simulink model "Dynamics_test1"  (R2021b)
settings: Solver=VariableStepAuto  StartTime=0.0  StopTime=10.0  RelTol=1e-3
InitFcn:
  | % ************** Initiate forces
  | % f0=[0;0;0;0;0;0];
  | % f0=[0;0;0;0;0;0;0];
  | f_0=[0;0;0];
  | f_m=[0;0];
  | f_e=[0;0;0;0;0;0];
  | % ************** Initiate states
  | q_m=[0;0];
  | q_dot_m=[0;0];
  | P=[0;0;0];
  | V_I0=[0;0;0];
  | % ************** Load main
  | %run(Main.m)
values from neighbouring files (symbols this model uses):
  diag_M = diagonalize(M_frak0, M_frak)    [Create_Robot.m]    (also in Main.m; diagonalize.m = zeros(6*(n+1),6*(n+1)); test_C_Main.m)
  iota0 = [1 0 0; 0 1 0;zeros(3,3);0 0 1]    [Create_Robot.m]    (also in Main.m = eye(6,6); test_C_Main.m)
  Xi_m_matrix = zeros(6*n,n)    [Create_Robot.m]    (also in Main.m; test_C_Main.m)
undefined symbols (not defined in the file or in its folder): Xi_m
settings Model: Creator=Bmmog  LastModifiedBy=Bmmog
settings SolverCC: AllowMultiTaskInputOutput=on

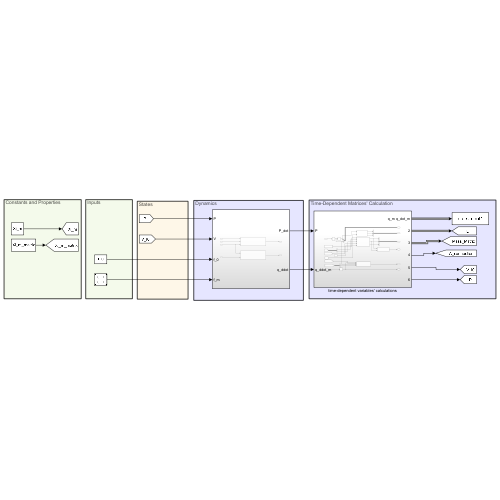
[thumbnail: Simulink's stored preview of the top-level diagram]
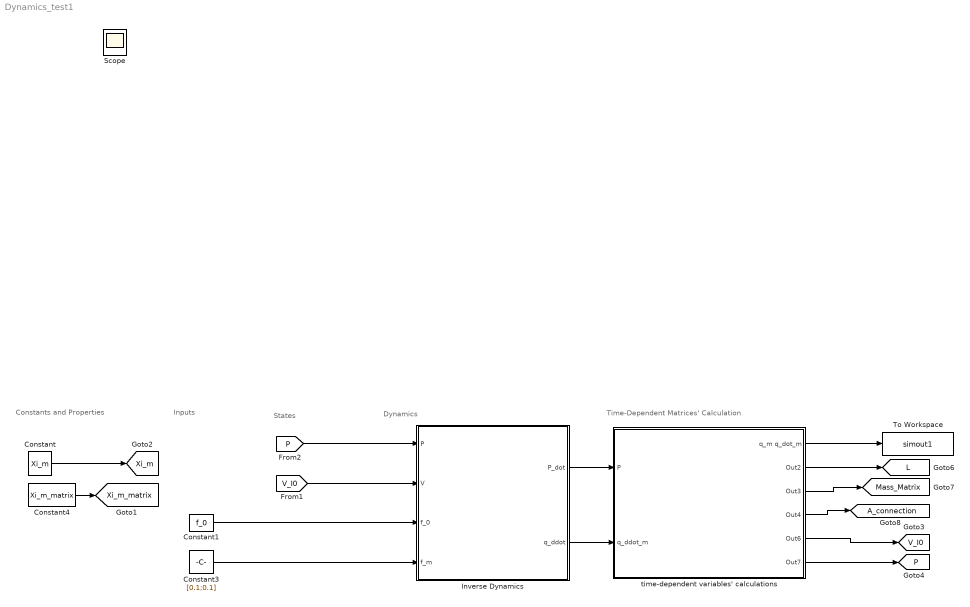
== system Dynamics_test1 ==
  note: Time-Dependent Matrices' Calculation
  note: States
  note: Inputs
  note: Dynamics
  note: Constants and Properties
  Constant : Constant  Value=Xi_m  VectorParams1D=off
  Constant1 : Constant  Value=f_0  VectorParams1D=off
  Constant3 : Constant  Value=[0.1;0.1]  VectorParams1D=off
  Constant4 : Constant  Value=Xi_m_matrix  VectorParams1D=off
  Inverse Dynamics : Subsystem
  To Workspace : ToWorkspace  VariableName=simout1  SaveFormat=Timeseries  SampleTime=-1
  time-dependent variables' calculations : Subsystem
  Scope : Scope
  tag scope: A_connection=global, L=global, Mass_Matrix=global, P=global, V_I0=global, Xi_m=global, Xi_m_matrix=global
  wires:
  Constant/1 -> [Xi_m]
  Constant4/1 -> [Xi_m_matrix]
  Constant1/1 -> Inverse Dynamics/3(f_0)
  Constant3/1 -> Inverse Dynamics/4(f_m)
  [P] -> Inverse Dynamics/1(P)
  [V_I0] -> Inverse Dynamics/2(V)
  time-dependent variables' calculations/6(Out7) -> [P]
  time-dependent variables' calculations/5(Out6) -> [V_I0]
  time-dependent variables' calculations/4(Out4) -> [A_connection]
  time-dependent variables' calculations/3(Out3) -> [Mass_Matrix]
  time-dependent variables' calculations/2(Out2) -> [L]
  time-dependent variables' calculations/1(q_m q_dot_m) -> To Workspace/1
  Inverse Dynamics/1(P_dot) -> time-dependent variables' calculations/1(P)
  Inverse Dynamics/2(q_ddot) -> time-dependent variables' calculations/2(q_ddot_m)

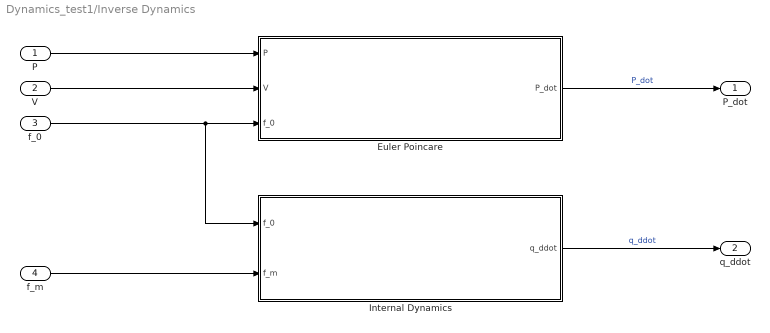
== system Dynamics_test1/Inverse Dynamics ==
  P : Inport
  V : Inport  Port=2
  f_0 : Inport  Port=3
  f_m : Inport  Port=4
  Euler Poincare : Subsystem
  Internal Dynamics : Subsystem
  P_dot : Outport
  q_ddot : Outport  Port=2
  wires:
  f_0/1 -> Internal Dynamics/1(f_0), Euler Poincare/3(f_0)
  f_m/1 -> Internal Dynamics/2(f_m)
  Internal Dynamics/1(q_ddot) -> q_ddot/1  "q_ddot"
  Euler Poincare/1(P_dot) -> P_dot/1  "P_dot"
  P/1 -> Euler Poincare/1(P)
  V/1 -> Euler Poincare/2(V)

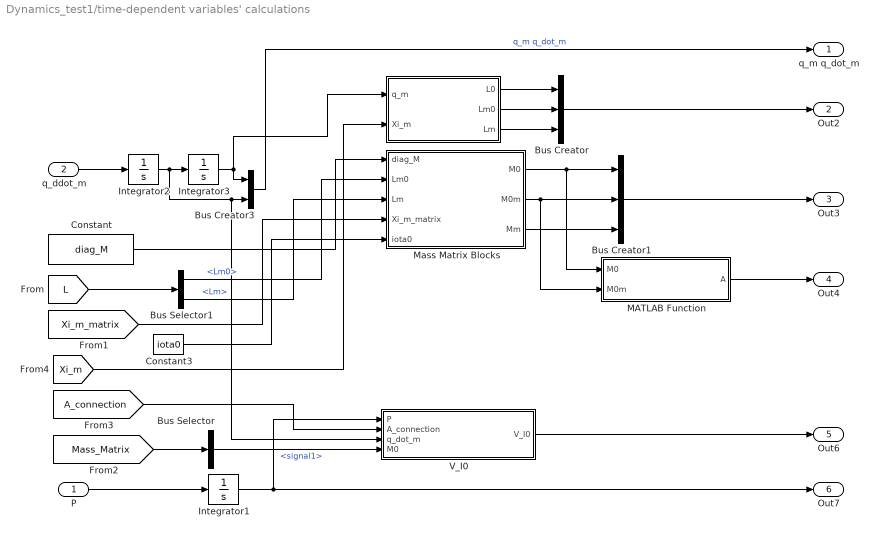
== system Dynamics_test1/time-dependent variables' calculations ==
  P : Inport
  q_ddot_m : Inport  Port=2
  " " : MATLAB Function  TreatAsAtomicUnit=on
  Bus Creator : BusCreator  Inputs=3
  Bus Creator1 : BusCreator  Inputs=3
  Bus Creator3 : BusCreator  Inputs=2
  Bus Selector : BusSelector  OutputSignals=signal1
  Bus Selector1 : BusSelector  OutputSignals=Lm0,Lm
  Constant : Constant  Value=diag_M  VectorParams1D=off
  Constant3 : Constant  Value=iota0  VectorParams1D=off
  Integrator1 : Integrator
  Integrator2 : Integrator
  Integrator3 : Integrator
  MATLAB Function : MATLAB Function  TreatAsAtomicUnit=on
  Mass Matrix Blocks : Subsystem
  V_I0 : MATLAB Function  TreatAsAtomicUnit=on
  q_m q_dot_m : Outport
  Out2 : Outport  Port=2
  Out3 : Outport  Port=3
  Out4 : Outport  Port=4
  Out6 : Outport  Port=5
  Out7 : Outport  Port=6
  wires:
  Mass Matrix Blocks/3(Mm) -> Bus Creator1/3
  Mass Matrix Blocks/2(M0m) -> MATLAB Function/2(M0m), Bus Creator1/2
  Integrator2/1 -> V_I0/3(q_dot_m), Bus Creator3/2, Integrator3/1
  Bus Creator3/1 -> q_m q_dot_m/1  "q_m q_dot_m"
  Mass Matrix Blocks/1(M0) -> MATLAB Function/1(M0), Bus Creator1/1
  Integrator1/1 -> Out7/1, V_I0/1(P)
  q_ddot_m/1 -> Integrator2/1
  V_I0/1(V_I0) -> Out6/1
  MATLAB Function/1(A) -> Out4/1
  Bus Creator1/1 -> Out3/1
  P/1 -> Integrator1/1
  " "/1(L0) -> Bus Creator/1
  " "/3(Lm) -> Bus Creator/3
  " "/2(Lm0) -> Bus Creator/2
  Bus Creator/1 -> Out2/1
  Constant3/1 -> Mass Matrix Blocks/5(iota0)
  Constant/1 -> Mass Matrix Blocks/1(diag_M)
  Bus Selector1/2 -> Mass Matrix Blocks/3(Lm)  "<Lm>"
  [Xi_m_matrix] -> Mass Matrix Blocks/4(Xi_m_matrix)
  Bus Selector1/1 -> Mass Matrix Blocks/2(Lm0)  "<Lm0>"
  [L] -> Bus Selector1/1
  [A_connection] -> V_I0/2(A_connection)
  Bus Selector/1 -> V_I0/4(M0)  "<signal1>"
  [Mass_Matrix] -> Bus Selector/1
  [Xi_m] -> " "/2(Xi_m)
  Integrator3/1 -> Bus Creator3/1, " "/1(q_m)

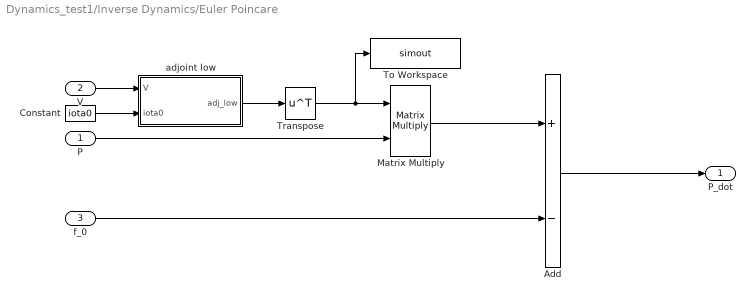
== system Dynamics_test1/Inverse Dynamics/Euler Poincare ==
  P : Inport
  V : Inport  Port=2
  f_0 : Inport  Port=3
  Add : Sum  Inputs=+-
  Constant : Constant  Value=iota0
  Matrix Multiply : Product  Multiplication=Matrix(*)
  To Workspace : ToWorkspace  VariableName=simout  SaveFormat=Timeseries  SampleTime=-1
  Transpose : Math  Operator=transpose  SaturateOnIntegerOverflow=on
  adjoint low : MATLAB Function  TreatAsAtomicUnit=on
  P_dot : Outport
  wires:
  P/1 -> Matrix Multiply/2
  adjoint low/1(adj_low) -> Transpose/1
  V/1 -> adjoint low/1(V)
  Transpose/1 -> To Workspace/1, Matrix Multiply/1
  Matrix Multiply/1 -> Add/1
  Add/1 -> P_dot/1
  f_0/1 -> Add/2
  Constant/1 -> adjoint low/2(iota0)

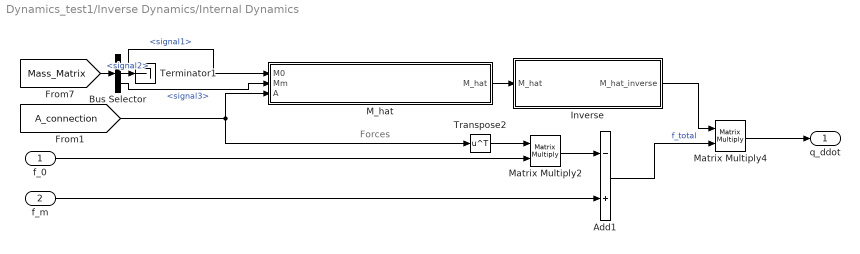
== system Dynamics_test1/Inverse Dynamics/Internal Dynamics ==
  note: Forces
  f_0 : Inport
  f_m : Inport  Port=2
  Add1 : Sum  Inputs=-+
  Bus Selector : BusSelector  OutputSignals=signal1,signal2,signal3
  Inverse : MATLAB Function  TreatAsAtomicUnit=on
  M_hat : MATLAB Function  TreatAsAtomicUnit=on
  Matrix Multiply2 : Product  Multiplication=Matrix(*)
  Matrix Multiply4 : Product  Multiplication=Matrix(*)
  Terminator1 : Terminator
  Transpose2 : Math  Operator=transpose  SaturateOnIntegerOverflow=on
  q_ddot : Outport
  wires:
  Add1/1 -> Matrix Multiply4/2  "f_total"
  Matrix Multiply2/1 -> Add1/1
  f_m/1 -> Add1/2
  Transpose2/1 -> Matrix Multiply2/1
  [A_connection] -> M_hat/3(A), Transpose2/1
  f_0/1 -> Matrix Multiply2/2
  Matrix Multiply4/1 -> q_ddot/1
  [Mass_Matrix] -> Bus Selector/1
  Bus Selector/1 -> M_hat/1(M0)  "<signal1>"
  Bus Selector/3 -> M_hat/2(Mm)  "<signal3>"
  M_hat/1(M_hat) -> Inverse/1(M_hat)
  Inverse/1(M_hat_inverse) -> Matrix Multiply4/1
  Bus Selector/2 -> Terminator1/1  "<signal2>"

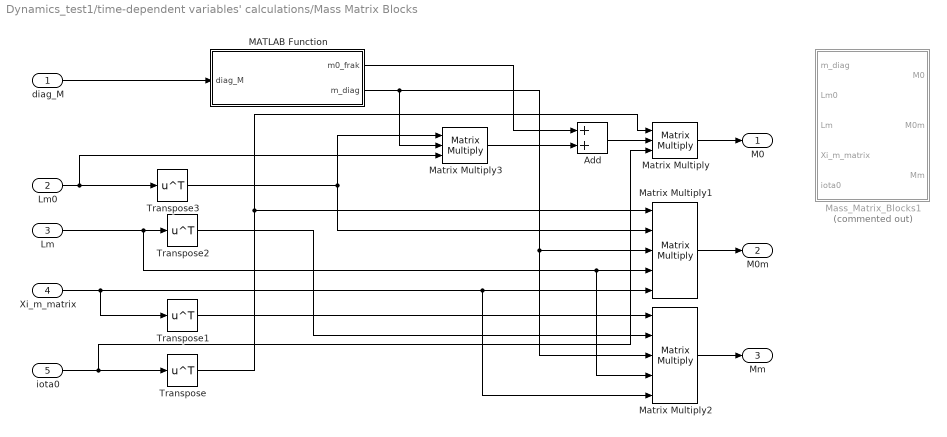
== system Dynamics_test1/time-dependent variables' calculations/Mass Matrix Blocks ==
  diag_M : Inport
  Lm0 : Inport  Port=2
  Lm : Inport  Port=3
  Xi_m_matrix : Inport  Port=4
  iota0 : Inport  Port=5
  Add : Sum
  MATLAB Function : MATLAB Function  TreatAsAtomicUnit=on
  Mass_Matrix_Blocks1 : MATLAB Function  Commented=on  TreatAsAtomicUnit=on
  Matrix Multiply : Product  Inputs=3  Multiplication=Matrix(*)
  Matrix Multiply1 : Product  Inputs=5  Multiplication=Matrix(*)
  Matrix Multiply2 : Product  Inputs=5  Multiplication=Matrix(*)
  Matrix Multiply3 : Product  Inputs=3  Multiplication=Matrix(*)
  Transpose{,1..3} (4 alike) : Math  Operator=transpose  SaturateOnIntegerOverflow=on
  M0 : Outport
  M0m : Outport  Port=2
  Mm : Outport  Port=3
  wires:
  Matrix Multiply2/1 -> Mm/1
  Xi_m_matrix/1 -> Transpose1/1, Matrix Multiply1/5, Matrix Multiply2/5
  Lm0/1 -> Matrix Multiply3/3, Transpose3/1
  Matrix Multiply/1 -> M0/1
  diag_M/1 -> MATLAB Function/1(diag_M)
  Matrix Multiply1/1 -> M0m/1
  iota0/1 -> Matrix Multiply/3, Transpose/1
  Lm/1 -> Matrix Multiply1/4, Matrix Multiply2/4, Transpose2/1
  Transpose/1 -> Matrix Multiply/1, Matrix Multiply1/1
  Transpose1/1 -> Matrix Multiply2/1
  Transpose2/1 -> Matrix Multiply2/2
  Transpose3/1 -> Matrix Multiply3/1, Matrix Multiply1/2
  MATLAB Function/2(m_diag) -> Matrix Multiply3/2, Matrix Multiply1/3, Matrix Multiply2/3
  MATLAB Function/1(m0_frak) -> Add/1
  Add/1 -> Matrix Multiply/2
  Matrix Multiply3/1 -> Add/2

== matlab function Dynamics_test1/Inverse Dynamics/Euler Poincare/adjoint low ==
  data: V input; adj_low output; iota0 input
function adj_low = adj_low(V, iota0)
% calculates the adjoint corresponding to the Lie bracket of vector V and ()
adj_low = adjoint_low(V,iota0);

== matlab function Dynamics_test1/Inverse Dynamics/Internal Dynamics/Inverse ==
  data: M_hat input; M_hat_inverse output
function M_hat_inverse = Inverse(M_hat)

M_hat_inverse=inv(M_hat);

== matlab function Dynamics_test1/Inverse Dynamics/Internal Dynamics/M_hat ==
  data: M0 input; Mm input; A input; M_hat output
function M_hat =M_hat(M0,Mm,A)
% Compute the Mass Matrix of the multibody system.
%   Input:
%   M0      Spacecraft mass matrix 
%   M0m     Coupling
%   Mm      Manipulator mass matrix

% Calculate M_hat
M_hat=Mm-transpose(A)*M0*A;


end

== matlab function Dynamics_test1/time-dependent variables' calculations/  ==
  data: q_m input; L0 output; Lm0 output; Lm output; Xi_m input
function [L0,Lm0,Lm] =L_calculator(q_m,Xi_m)
% Calculates the time-dependent L matrix
n=length(q_m);
L=zeros(6*(n+1),6*(n+1));
% Compute M_frak for ith body
% Calculate L matrix
for i=1:n
    for j=1:n
        if i>j
            Ad_temp=eye(6);
            for k=i:j
                Ad_temp=Ad_temp*Adjoint(g_Matrix(-Xi_m(:,k),q_m(k)));
            end
            L(6*(i-1)+1:6*(i-1)+6,6*(j-1)+1:6*(j-1)+6)=Ad_temp;
        elseif i==j
            L(6*(i-1)+1:6*(i-1)+6,6*(j-1)+1:6*(j-1)+6)=eye(6);
        elseif i<j
            L(6*(i-1)+1:6*(i-1)+6,6*(j-1)+1:6*(j-1)+6)=zeros(6);
        end
    end
end

L0=L(1:6,1:6);
Lm0=L(7:end,1:6);
Lm=L(7:end,7:end);

end

== matlab function Dynamics_test1/time-dependent variables' calculations/MATLAB Function ==
  data: M0 input; M0m input; A output
function A=A_connection(M0,M0m)
% Compute the connection A from mass properties

A=M0\M0m;

== matlab function Dynamics_test1/time-dependent variables' calculations/Mass Matrix Blocks/MATLAB Function ==
  data: diag_M input; m0_frak output; m_diag output
function [m0_frak,m_diag]=m_frak_decomp(diag_M)
% Compute the Mass Matrix of the multibody system.
%   Output:
%   M0      Spacecraft mass matrix 
%   M0m
%   Mm      Manipulator mass matrix

%n=length(q_m);

m0_frak=diag_M(1:6,1:6);
m_diag=diag_M(7:end,7:end);

== matlab function Dynamics_test1/time-dependent variables' calculations/Mass Matrix Blocks/Mass_Matrix_Blocks1 ==
  data: m_diag input; Lm0 input; Lm input; Xi_m_matrix input; M0 output; M0m output; Mm output; iota0 input
function [M0,M0m,Mm]=Mass_Matrix(m_diag,Lm0,Lm,Xi_m_matrix,iota0)
% Compute the Mass Matrix of the multibody system.
%   Output:
%   M0      Spacecraft mass matrix 
%   M0m
%   Mm      Manipulator mass matrix

%n=length(q_m);

m0_frak=m_diag(1:6,1:6);
m_diag=m_diag(7:end,7:end);

%Initiate
M0=[I0,zeros(3,3);zeros(3,3),m0*eye(3)];
M0m=zeros(6,6*n);
Mm=zeros(6*n,6*n);

%calculate transposes
iota0T=transpose(iota0);
Lm0T=transpose(Lm0);
LmT=transpose(Lm);
Xi_mT=transpose(Xi_m_matrix);

% Vehicle Spacecraft Mass matrix block
M0=iota0T*(m0_frak+Lm0T*m_diag*Lm0)*iota0;

% Vehicle Spacecraft Mass matrix block
M0m=iota0T*Lm0T*m_diag*Lm*Xi_m_matrix;

% Vehicle Spacecraft Mass matrix block
Mm=Xi_mT*LmT*m_diag*Lm*Xi_m_matrix;



end

== matlab function Dynamics_test1/time-dependent variables' calculations/V_I0 ==
  data: P input; A_connection input; q_dot_m input; M0 input; V_I0 output
function V_I0=V_I0(P,A_connection,q_dot_m,M0)
% Find the spaccecraft velocity V_I0
M0_inv=inv(M0);
% temp=P-transpose(A_connection)*q_dot_m;
V_I0=M0_inv\P-A_connection*q_dot_m;
